simulink model "robotics_2axis_PD_test"  (R2022a)
settings: Solver=VariableStepAuto  StartTime=0.0  StopTime=10.0  RelTol=1e-3
settings Model: Creator=user0612  LastModifiedBy=user0612

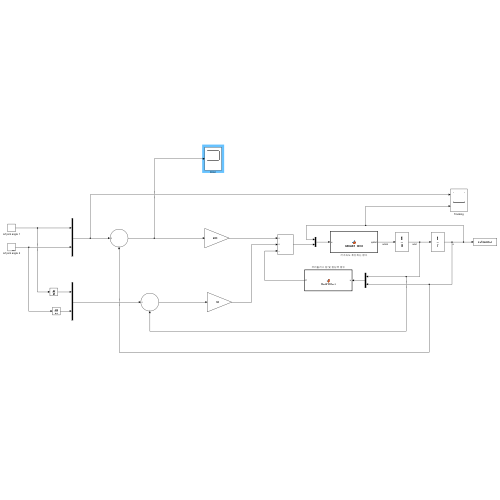
[thumbnail: Simulink's stored preview of the top-level diagram]
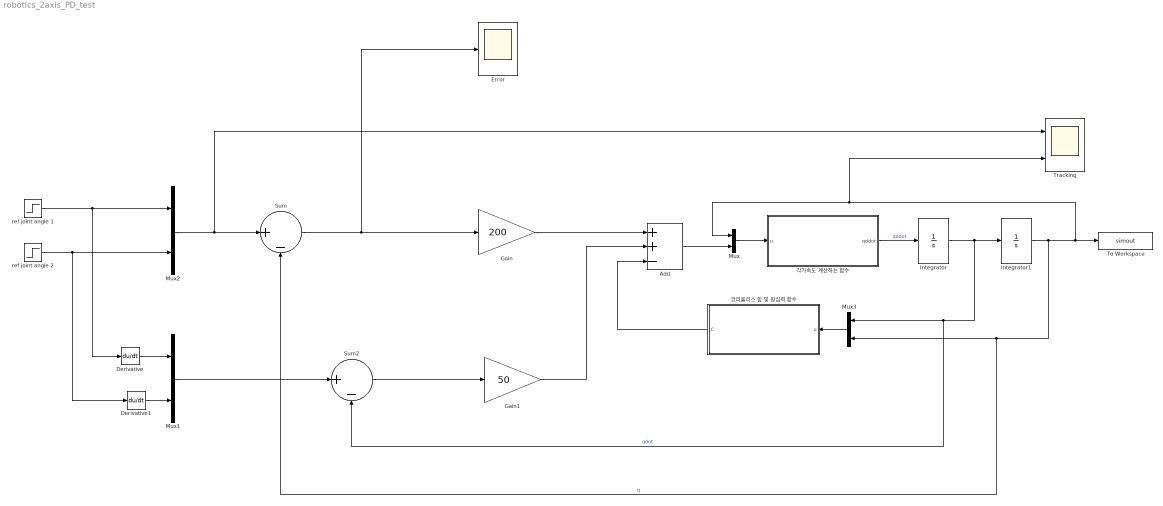
== system robotics_2axis_PD_test ==
  Add : Sum  Inputs=++-
  Derivative : Derivative
  Derivative1 : Derivative
  Error : Scope
  Gain : Gain  Gain=200
  Gain1 : Gain  Gain=50
  Integrator : Integrator  InitialCondition=zeros(2,1)
  Integrator1 : Integrator  InitialCondition=zeros(2,1)
  Mux{,1..3} (4 alike) : Mux  Inputs=2
  Sum : Sum  Inputs=|+-
  Sum2 : Sum  Inputs=|+-
  To Workspace : ToWorkspace  VariableName=simout  SaveFormat=Timeseries  SampleTime=-1
  Tracking : Scope  NumInputPorts=2
  ref joint angle 1 : Step  Time=0  Before=pi/4  After=pi/2  SampleTime=0
  ref joint angle 2 : Step  Time=0  Before=-pi/4  After=-pi/2  SampleTime=0
  각가속도 계산하는 함수 : MATLAB Function  TreatAsAtomicUnit=on
  코리올리스 힘 및 원심력 함수 : MATLAB Function  TreatAsAtomicUnit=on
  wires:
  ref joint angle 1/1 -> Mux2/1, Derivative/1
  Derivative/1 -> Mux1/1
  Sum/1 -> Error/1, Gain/1
  Gain/1 -> Add/1
  각가속도 계산하는 함수/1(qddot) -> Integrator/1  "qddot"
  Mux3/1 -> 코리올리스 힘 및 원심력 함수/1(u)
  코리올리스 힘 및 원심력 함수/1(C) -> Add/3
  Add/1 -> Mux/2
  Mux2/1 -> Tracking/1, Sum/1
  Integrator/1 -> Sum2/2, Mux3/1, Integrator1/1  "qdot"
  Mux1/1 -> Sum2/1
  Integrator1/1 -> Tracking/2, Mux/1, To Workspace/1, Sum/2, Mux3/2  "q"
  Sum2/1 -> Gain1/1
  Derivative1/1 -> Mux1/2
  ref joint angle 2/1 -> Derivative1/1, Mux2/2
  Gain1/1 -> Add/2
  Mux/1 -> 각가속도 계산하는 함수/1(u)

== matlab function robotics_2axis_PD_test/각가속도 계산하는 함수 ==
  data: u input; qddot output
function qddot = calculate_qddot(u) % u에는 q1, q2, q

m1 = 5; m2 = 5; l1 = 0.4; l2 = 0.4;

q1 = u(1); q2 = u(2);

% 관성행렬 성분 정의
d11 = (m1 + m2) * l1^2 + m2 * l2^2 + 2 * m2 * l1 * l2 * cos(q2);
d12 = m2 * l2^2 + m2 * l1 * l2 * cos(q2);
d21 = m2 * l2^2 + m2 * l1 * l2 * cos(q2);
d22 = m2 * l2^2;

% 관성행렬
D = [d11 d12; d21 d22];

% 관성행렬 역행렬
D_inv = inv(D);

tau_minus_C = [u(3); u(4)];

qddot = (D_inv * tau_minus_C);

end

== matlab function robotics_2axis_PD_test/코리올리스 힘 및 원심력 함수 ==
  data: u input; C output
% u에는 qdot1, qdot2, q1, q2
function C = CorANDCent(u) 

qdot1 = u(1); qdot2 = u(2); q1 = u(3); q2 = u(4);
m1 = 5; m2 = 5; l1 = 0.4; l2 = 0.4;

% 코리올리스 및 관성력 행렬 성분
C1 = -m2 * l1 * l2 * sin(q2) * (2 * qdot1 * qdot2 + qdot2^2);
C2 = m2 * l1 * l2 * qdot1^2 * sin(q2);

% 코리올리스 및 관성력 행렬
C = [C1; C2];

end
